simulink model "flipFlopMove"  (R2018b)
settings: Solver=ode3  StartTime=0.0  StopTime=10  RelTol=1e-3  EnableMultiTasking=on
libraries: legoev3lib x3
settings Model: FPTRunName=Active  ExtModeTrigDuration=2  Creator=svdh  LastModifiedBy=svdh
settings SolverCC: PositivePriorityOrder=on
settings DataIOCC: LimitDataPoints=on  SaveFormat=Array
settings OptimizationCC: ExpressionDepthLimit=2147483647  LifeSpan=Inf  MaxStackSize=64
settings DebuggingCC: UnderspecifiedInitializationDetection=Classic  MergeDetectMultiDrivingBlocksExec=none  FcnCallInpInsideContextMsg=warning  AllowSymbolicDim=off  StateNameClashWarn=warning  SFUnexpectedBacktrackingDiag=warning  SFNoUnconditionalDefaultTransitionDiag=warning  SFExecutionAtInitializationDiag=none
settings HardwareCC: ProdBitPerPointer=32  ProdBitPerSizeT=32  ProdBitPerPtrDiffT=32  ProdLargestAtomicInteger=Long  ProdWordSize=32  ProdHWDeviceType=ARM Compatible->ARM 9  UseEmbeddedCoderFeatures=off
settings ModelReferenceCC: PropagateSignalLabelsOutOfModel=off
settings SFSimCC: SimUseLocalCustomCode=off
settings RTWCC: SystemTargetFile=ert.tlc  HardwareBoard=LEGO MINDSTORMS EV3  TemplateMakefile=ert_default_tmf  GenerateReport=on  RTWVerbose=off  RTWUseLocalCustomCode=off  Toolchain=Sourcery G++ Lite v2009q3  BuildConfiguration=Faster Runs  LaunchReport=on
settings CodeAppCC: ForceParamTrailComments=on  OperatorAnnotations=on  StateflowObjectComments=on  MATLABSourceComments=on
settings ERTTargetCC: MultiwordLength=2048  ERTCustomFileBanners=off  SupportContinuousTime=on  SupportNonInlinedSFcns=on  RemoveResetFunc=off  SupportVariableSizeSignals=on  ModelStepFunctionPrototypeControlCompliant=off
settings ConfigComp: CovMetricSettings=dw  CovHtmlReporting=on  CovSaveCumulativeToWorkspaceVar=on  CovSaveSingleToWorkspaceVar=on  CovExternalEMLEnable=off  CovSFcnEnable=off

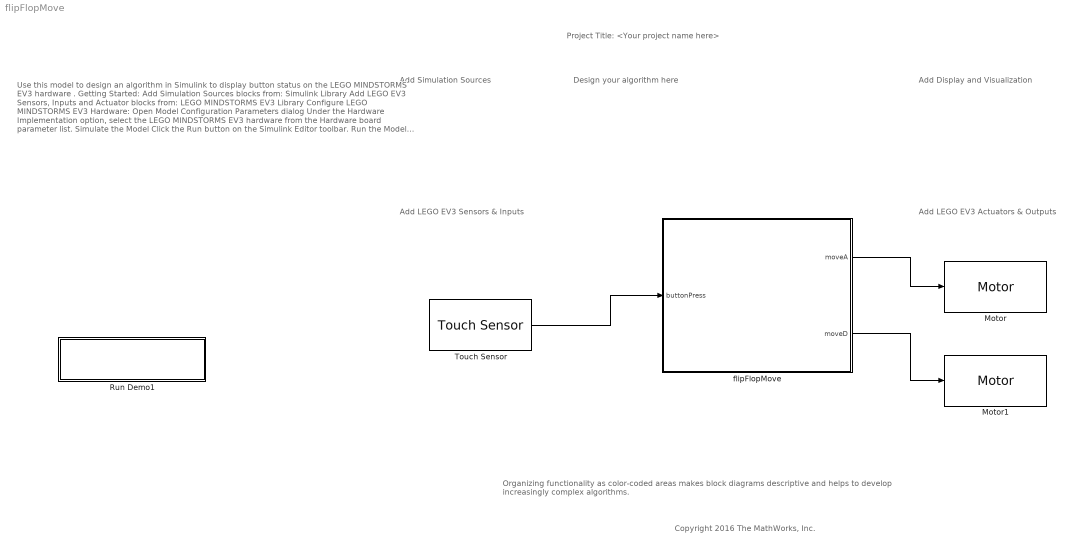
== system flipFlopMove ==
  note: Project Title: <Your project name here>
  note: Copyright 2016 The MathWorks, Inc.
  note: Add LEGO EV3 Sensors & Inputs
  note: Add LEGO EV3 Actuators & Outputs
  note: Add Display and Visualization
  note: Design your algorithm here
  note: Add Simulation Sources
  note: Use this model to design an algorithm in Simulink to display button status on the LEGO MINDSTORMS EV3 hardware .
      |
      | Getting Started:
      |
      | Add Simulation Sources blocks from:
      | Simulink Library
      | Add LEGO EV3 Sensors, Inputs and Actuator blocks from:
      | LEGO MINDSTORMS EV3 Library
      |
      | Configure LEGO MINDSTORMS EV3 Hardware:
      |
      | Open Model Configuration Parameters dialog
      | Under the Hardware Implementation option, select the LEGO MINDSTORMS EV3 hardware from the Hardware board parameter list.
      |
      | Simulate the Model
      |
      | Click the Run button on the Simulink Editor toolbar.
      |
      | Run the Model on LEGO MINDSTORMS EV3 Hardware
      |
      | Click the Deploy to Hardware button on the Simulink Editor toolbar.
      |
      | Other Things to Try:
      |
      | Create and run a model that detects the obstacle and stops the LEGO EV3 robot. HINT: Use Ultrasonic Sensor and Motor blocks.
  note: Organizing functionality as color-coded areas makes block diagrams descriptive and helps to develop increasingly complex algorithms.
  Motor : legoev3lib/Motor  sportNumber=A  sstopAction=Brake
  Motor1 : legoev3lib/Motor  sportNumber=D  sstopAction=Brake
  Run Demo1 : Subsystem  Description=Controls host-side RTDX processing.
      mask Display: pic=imread('ev3DeploytoHardware.png');image(pic);
  Touch Sensor : legoev3lib/Touch Sensor  portNumber=1  sampleTime=0.1
      settings: SourceProductName=Simulink Support Package for LEGO MINDSTORMS EV3 Hardware  SourceProductBaseCode=LEGOEV3
  flipFlopMove : Stateflow chart  TreatAsAtomicUnit=on
  wires:
  Touch Sensor/1 -> flipFlopMove/1(buttonPress)
  flipFlopMove/1(moveA) -> Motor/1
  flipFlopMove/2(moveD) -> Motor1/1

== system flipFlopMove/Run Demo1 ==

== stateflow chart flipFlopMove/flipFlopMove ==
  state Waiting1
  state Moving
    entry:
    moveA = 100
    moveD = 100
  state Stopped
    entry:
    moveA = 0
    moveD = 0
  state Waiting
  (default) -> Waiting1
  Waiting1 -> Moving : [buttonPress == 1]
  Stopped -> Waiting1 : [buttonPress == 0]
  Moving -> Waiting : [buttonPress == 0]
  Waiting -> Stopped : [buttonPress == 1]
  data: buttonPress input; moveA output; moveD output
